simulink model "manipulator_cl"  (R2018b)
settings: Solver=ode45  StartTime=0.0  StopTime=5  RelTol=1e-9
values from neighbouring files (symbols this model uses):
  sys_phode = ss(J_ode * Q_ode, B_ode, B_ode'* Q_ode, 0)    [ph_model.m]
undefined symbols (not defined in the file or in its folder): alpha_rel, kp1, kp2, kv1, kv2, rad_deg
settings Model: Creator=a.brugnoli  LastModifiedBy=a.brugnoli

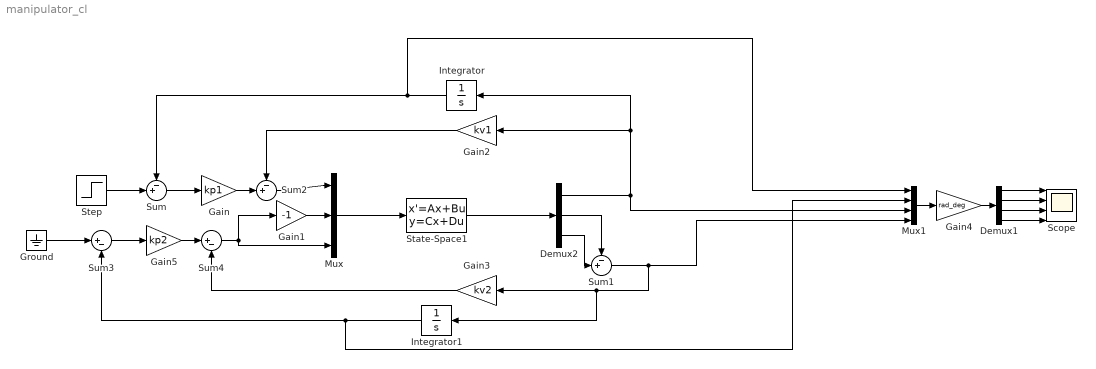
== system manipulator_cl ==
  Demux1 : Demux
  Demux2 : Demux  Outputs=3
  Gain : Gain  Gain=kp1
  Gain1 : Gain  Gain=-1
  Gain2 : Gain  Gain=kv1
  Gain3 : Gain  Gain=kv2
  Gain4 : Gain  Gain=rad_deg
  Gain5 : Gain  Gain=kp2
  Ground : Ground
  Integrator : Integrator
  Integrator1 : Integrator
  Mux : Mux  Inputs=3
  Mux1 : Mux
  Scope : Scope  NumInputPorts=4
  State-Space1 : StateSpace  A=sys_phode.A  B=sys_phode.B  C=sys_phode.C  D=sys_phode.D  InitialCondition=0
  Step : Step  After=alpha_rel  SampleTime=0
  Sum : Sum  Inputs=-+|
  Sum1 : Sum  Inputs=-+|
  Sum2 : Sum  Inputs=-+|
  Sum3 : Sum  Inputs=|+-
  Sum4 : Sum  Inputs=|+-
  wires:
  State-Space1/1 -> Demux2/1
  Gain2/1 -> Sum2/1
  Integrator/1 -> Mux1/1, Sum/1
  Step/1 -> Sum/2
  Gain/1 -> Sum2/2
  Sum/1 -> Gain/1
  Demux1/1 -> Scope/1
  Mux1/1 -> Gain4/1
  Demux2/1 -> Mux1/3, Gain2/1, Integrator/1
  Gain4/1 -> Demux1/1
  Demux1/4 -> Scope/4
  Demux1/3 -> Scope/3
  Demux1/2 -> Scope/2
  Mux/1 -> State-Space1/1
  Sum2/1 -> Mux/1
  Ground/1 -> Sum3/1
  Gain5/1 -> Sum4/1
  Gain3/1 -> Sum4/2
  Sum3/1 -> Gain5/1
  Demux2/3 -> Sum1/2
  Demux2/2 -> Sum1/1
  Sum4/1 -> Mux/3, Gain1/1
  Sum1/1 -> Integrator1/1, Gain3/1, Mux1/4
  Integrator1/1 -> Mux1/2, Sum3/2
  Gain1/1 -> Mux/2
